simulink model "Radiator_version_4"  (R2023b)
settings: Solver=VariableStepAuto  StartTime=0.0  StopTime=1697  RelTol=1e-3
undefined symbols (not defined in the file or in its folder): _speed, Endurance
settings Model: Creator=minho  LastModifiedBy=minho

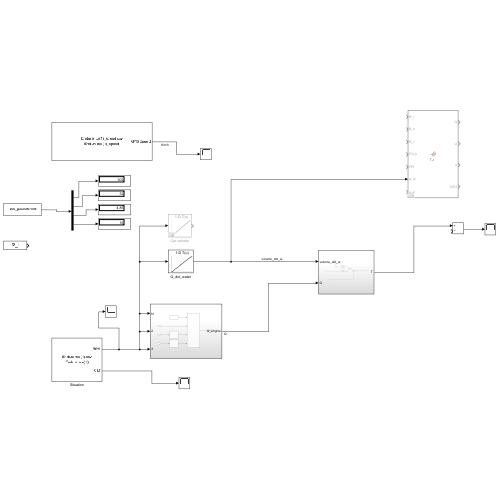
[thumbnail: Simulink's stored preview of the top-level diagram]
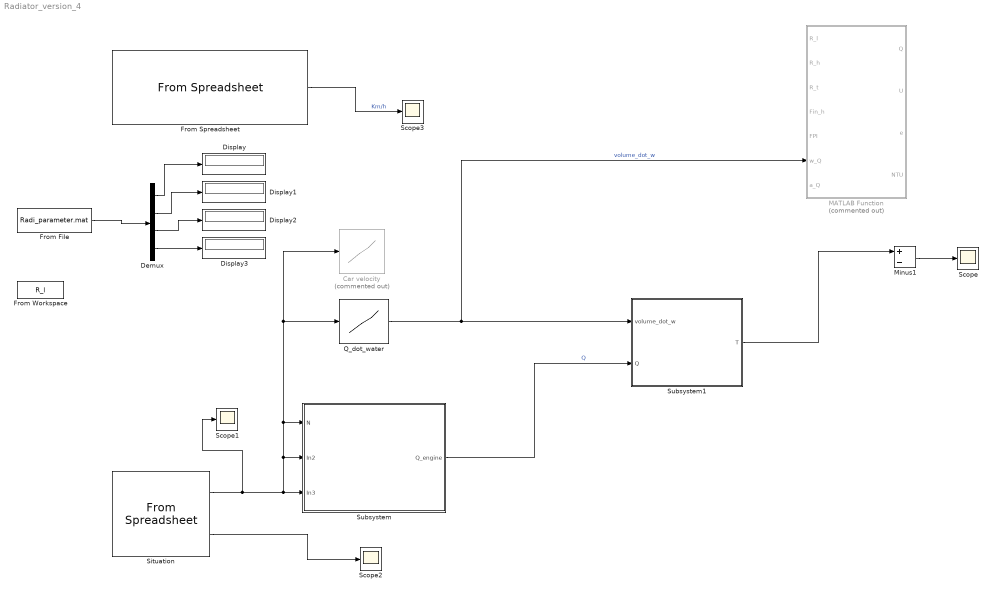
== system Radiator_version_4 ==
  Car velocity : Lookup_n-D  Commented=on  NumberOfTableDimensions=1  BreakpointsForDimension1=|  Table=|  InternalRulePriority=Speed  RndMeth=Simplest
      BreakpointsForDimension1=|
      | [2500
      | 3000
      | 3500
      | 4000
      | 4500
      | 5000
      | 5500
      | 6000
      | 6500
      | 7000
      | 7500
      | 8000
      | 8500
      | 9000
      | 9500
      | 10000
      | 10500
      | 11000
      | 11500
      | 12000
      | ]
      Table=|
      | [14.74651903
      | 17.69582284
      | 20.64512664
      | 23.59443045
      | 26.54373425
      | 29.49303806
      | 32.44234187
      | 35.39164567
      | 38.34094948
      | 41.29025329
      | 44.23955709
      | 47.1888609
      | 50.1381647
      | 53.08746851
      | 56.03677232
      | 58.98607612
      | 61.93537993
      | 64.88468373
      | 67.83398754
      | 70.78329135
      | ]
  Demux : Demux
  Display{,1..3} (4 alike) : Display
  From Workspace : FromWorkspace  VariableName=R_l
  From File : FromFile  FileName=Radi_parameter.mat  SampleTime=0
  From Spreadsheet : FromSpreadsheet  FileName=Endurance(1)_speed.csv  SheetName=Endurance(1)_speed
  MATLAB Function : MATLAB Function  Commented=on  TreatAsAtomicUnit=on
  Minus1 : Sum  Inputs=+-
  Q_dot_water : Lookup_n-D  NumberOfTableDimensions=1  BreakpointsForDimension1=|  Table=|  InternalRulePriority=Speed  RndMeth=Simplest
      BreakpointsForDimension1=|
      | [2000
      | 2500
      | 3000
      | 3500
      | 4000
      | 4500
      | 5000
      | 5500
      | 6000
      | 6500
      | 7000
      | 7500
      | 8000
      | 8500
      | 9000
      | 9500
      | 10000
      | 10500
      | 11000
      | 11500
      | 12000
      | ]
      Table=|
      | [0.000204
      | 0.000255
      | 0.000306
      | 0.000357
      | 0.000408
      | 0.000459
      | 0.00051
      | 0.000561
      | 0.000612
      | 0.000663
      | 0.000714
      | 0.000765
      | 0.000816
      | 0.000867
      | 0.000918
      | 0.000969
      | 0.001021
      | 0.001072
      | 0.001123
      | 0.001174
      | 0.001225
      | ]
  Scope{,1..3} (4 alike) : Scope
  Situation : FromSpreadsheet  FileName=Endurance(1).csv  SheetName=Endurance(1)
  Subsystem : Subsystem
  Subsystem1 : Subsystem
  wires:
  Situation/1 -> Scope1/1, Subsystem/3(In3), Car velocity/1, Q_dot_water/1, Subsystem/1(N), Subsystem/2(In2)
  Situation/2 -> Scope2/1
  Q_dot_water/1 -> MATLAB Function/6(w_Q), Subsystem1/1(volume_dot_w)  "volume_dot_w"
  Subsystem/1(Q_engine) -> Subsystem1/2(Q)  "Q"
  Subsystem1/1(T) -> Minus1/1
  Minus1/1 -> Scope/1
  From Spreadsheet/1 -> Scope3/1  "Km/h"
  From File/1 -> Demux/1
  Demux/1 -> Display/1
  Demux/2 -> Display1/1
  Demux/3 -> Display2/1
  Demux/4 -> Display3/1

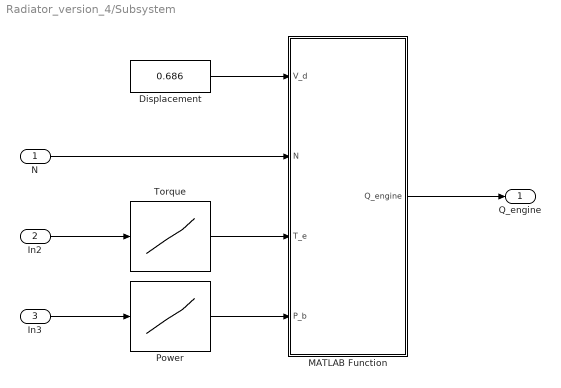
== system Radiator_version_4/Subsystem ==
  N : Inport
  In2 : Inport  Port=2
  In3 : Inport  Port=3
  Displacement : Constant  Value=0.686
  MATLAB Function : MATLAB Function  TreatAsAtomicUnit=on
  Power : Lookup_n-D  NumberOfTableDimensions=1  BreakpointsForDimension1=|  Table=|  InternalRulePriority=Speed  RndMeth=Simplest
      BreakpointsForDimension1=|
      | [2000
      | 2500
      | 3000
      | 3500
      | 4000
      | 4500
      | 5000
      | 5500
      | 6000
      | 6500
      | 7000
      | 7500
      | 8000
      | 8500
      | 9000
      | 9500
      | 10000
      | 10500]
      Table=|
      | [8.21009535654529
      | 12.6810277191857
      | 17.1341120484423
      | 21.2391597267150
      | 25.7011680726635
      | 27.6287556781133
      | 31.2340584216397
      | 35.3391060999123
      | 39.0657754704486
      | 43.2307925408908
      | 46.4762789313999
      | 49.1213574788781
      | 49.3462426995140
      | 50.9739833441160
      | 52.1990723555796
      | 50.8668951438132
      | 46.1193182637240
      | 41.9785745186837]
  Torque : Lookup_n-D  NumberOfTableDimensions=1  BreakpointsForDimension1=|  Table=|  InternalRulePriority=Speed  RndMeth=Simplest
      BreakpointsForDimension1=|
      | [2000
      | 2500
      | 3000
      | 3500
      | 4000
      | 4500
      | 5000
      | 5500
      | 6000
      | 6500
      | 7000
      | 7500
      | 8000
      | 8500
      | 9000
      | 9500
      | 10000
      | 10500]
      Table=|
      | [39.2003177775000
      | 48.4379578798500
      | 54.5395725600000
      | 57.9482958450000
      | 61.3570191300000
      | 58.6300405020000
      | 59.6526574875000
      | 61.3570191300000
      | 62.1751127184000
      | 63.5113322461200
      | 63.4022531010000
      | 62.5432548331800
      | 58.9027383648000
      | 57.2665511880000
      | 55.3849359346800
      | 51.1308492750000
      | 44.0407048422000
      | 38.1777007920000]
  Q_engine : Outport
  wires:
  MATLAB Function/1(Q_engine) -> Q_engine/1
  N/1 -> MATLAB Function/2(N)
  Power/1 -> MATLAB Function/4(P_b)
  Torque/1 -> MATLAB Function/3(T_e)
  In2/1 -> Torque/1
  Displacement/1 -> MATLAB Function/1(V_d)
  In3/1 -> Power/1

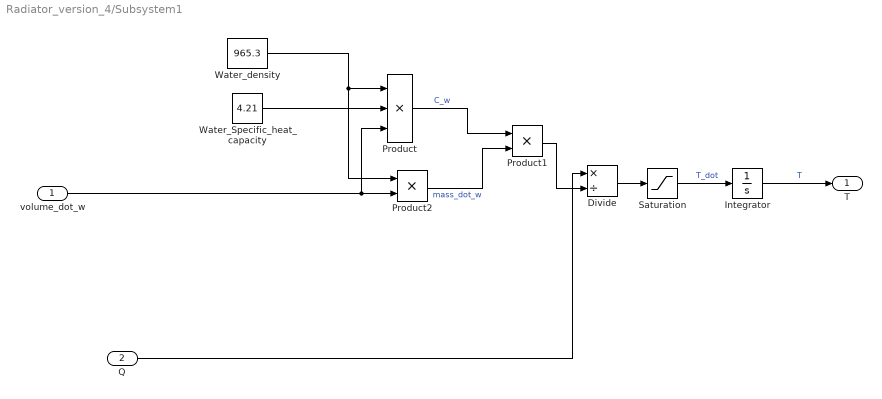
== system Radiator_version_4/Subsystem1 ==
  volume_dot_w : Inport
  Q : Inport  Port=2
  Divide : Product  Inputs=*/
  Integrator : Integrator  InitialCondition=43
  Product : Product  Inputs=3
  Product1 : Product
  Product2 : Product
  Saturation : Saturate  UpperLimit=1000  LowerLimit=0
  Water_Specific_heat_capacity : Constant  Value=4.21
  Water_density : Constant  Value=965.3
  T : Outport
  wires:
  Product2/1 -> Product1/2  "mass_dot_w"
  Water_Specific_heat_capacity/1 -> Product/2
  Water_density/1 -> Product/1, Product2/1
  Product1/1 -> Divide/2
  Divide/1 -> Saturation/1
  volume_dot_w/1 -> Product2/2, Product/3
  Product/1 -> Product1/1  "C_w"
  Saturation/1 -> Integrator/1  "T_dot"
  Q/1 -> Divide/1
  Integrator/1 -> T/1  "T"

== matlab function Radiator_version_4/MATLAB Function ==
  data: R_l input; Q output; R_h input; R_t input; Fin_h input; FPI input; w_Q input; a_Q input; U output; e output; NTU output
function [Q,U,e,NTU] = fcn(R_l,R_h,R_t,Fin_h,FPI,w_Q,a_Q)

[Q,U,e,NTU] = RadiCalculator(R_l,R_h,R_t,Fin_h,FPI,w_Q,a_Q);

end

== matlab function Radiator_version_4/Subsystem/MATLAB Function ==
  data: V_d input; Q_engine output; N input; T_e input; P_b input
function Q_engine = Lahivc(V_d, N, T_e, P_b)

% Lahivc Function from Ford

Q_engine = (8.66*V_d*N+108.93*T_e+1119.74*P_b-1010*V_d+2890)/3412.2;
